simulink model "dynamics_kinematics"  (Simulink 7.9)
settings: Solver=ode15s  StartTime=0.0  StopTime=10.0  RelTol=1e-3
values from neighbouring files (symbols this model uses):
  current_s = [0,1,0,0,0,0, 0,0,0,0,0,0] * 0    [kinematic_parameters.m]
  initial_ee_eta = zeros(1,6)    [kinematic_parameters.m]
  initial_eta = [0,0,0,0,0,0]    [kinematic_parameters.m]
  initial_q = [0,65*d2r,-(65+90)*d2r,90*d2r,-90*d2r,0]    [kinematic_parameters.m]
  inner_motion_vec = [0,0,0,0,0,1,0,0,0,0,0,0]    [kinematic_parameters.m]
  K_i = diag([1,1,1,1,1,1,   1,1,1,1,1,1])*0.5 * 0    [kinematic_parameters.m]
  K_p = diag([1,1,1,1,1,1,   1,1,1,1,1,1])    [kinematic_parameters.m]
  v_ee_c = [0.1,0,0,0,0,0]    [kinematic_parameters.m]
libraries: simulink x1
settings Model: Creator=simena  LastModifiedBy=simena  SimulationMode=accelerator
settings OptimizationCC: EfficientMapNaN2IntZero=off
settings HardwareCC: TargetIntDivRoundTo=Zero  TargetEndianess=LittleEndian  TargetHWDeviceType=MATLAB Host  ProdEqTarget=off
settings CodeAppCC: MaxIdLength=128
settings GRTTargetCC: CombineOutputUpdateFcns=off  GRTInterface=on

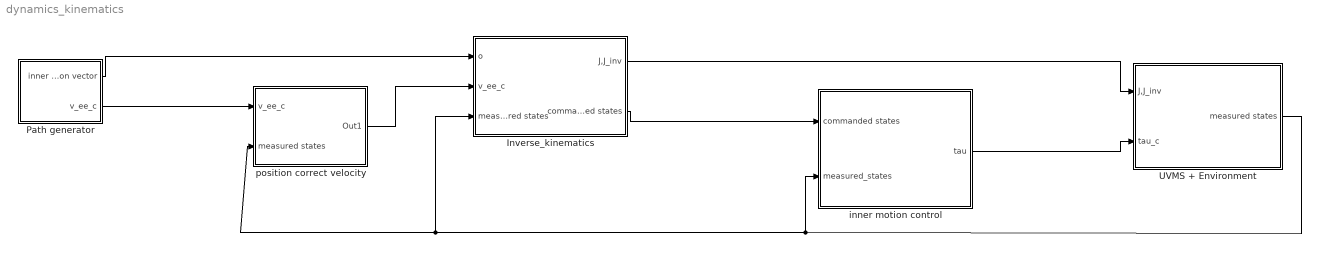
== system dynamics_kinematics ==
  "Inverse_kinematics " : Subsystem
  Path generator : Subsystem
  UVMS + Environment : Subsystem
  inner motion control : Subsystem
  position correct velocity : Subsystem
  wires:
  inner motion control/1(tau) -> UVMS + Environment/2(tau_c)
  UVMS + Environment/1(measured states) -> inner motion control/2(measured_states), "Inverse_kinematics "/3(measured states), position correct velocity/2(measured states)
  "Inverse_kinematics "/2(commanded states) -> inner motion control/1(commanded states)
  Path generator/1(inner motion vector) -> "Inverse_kinematics "/1(o)
  Path generator/2(v_ee_c) -> position correct velocity/1(v_ee_c)
  position correct velocity/1(Out1) -> "Inverse_kinematics "/2(v_ee_c)
  "Inverse_kinematics "/1(J,J_inv) -> UVMS + Environment/1(J,J_inv)

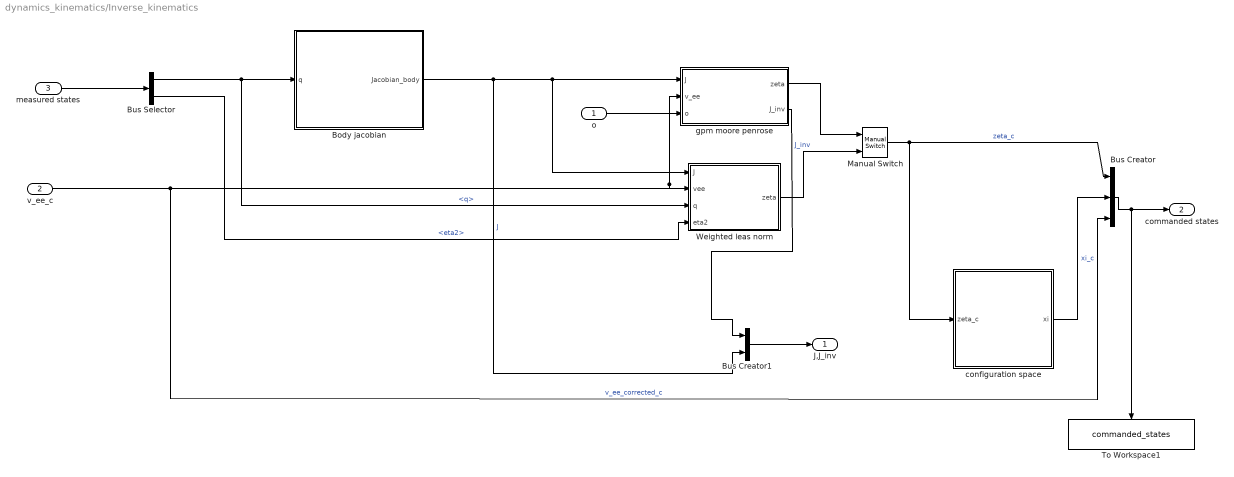
== system dynamics_kinematics/Inverse_kinematics  ==
  o : Inport
  v_ee_c : Inport  Port=2
  measured states : Inport  Port=3
  Body jacobian : MATLAB Function  TreatAsAtomicUnit=on
  Bus Creator : BusCreator  Inputs=3
  Bus Creator1 : BusCreator  Inputs=2
  Bus Selector : BusSelector  OutputSignals=xi.q,xi.eta2
  Manual Switch : simulink/Signal Routing/Manual Switch  sw=0  action=0  varsize=off
  To Workspace1 : ToWorkspace  VariableName=commanded_states  SampleTime=-1  SaveFormat=Timeseries
  Weighted leas norm : MATLAB Function  TreatAsAtomicUnit=on
  configuration space : Subsystem
  gpm moore penrose : Subsystem
  J,J_inv : Outport
  commanded states : Outport  Port=2
  wires:
  gpm moore penrose/1(zeta) -> Manual Switch/1
  Weighted leas norm/1(zeta) -> Manual Switch/2
  Manual Switch/1 -> configuration space/1(zeta_c), Bus Creator/1  "zeta_c"
  measured states/1 -> Bus Selector/1
  Bus Selector/1 -> Body jacobian/1(q), Weighted leas norm/3(q)  "<q>"
  Body jacobian/1(Jacobian_body) -> gpm moore penrose/1(J), Weighted leas norm/1(J), Bus Creator1/2  "J"
  Bus Selector/2 -> Weighted leas norm/4(eta2)  "<eta2>"
  v_ee_c/1 -> gpm moore penrose/2(v_ee), Weighted leas norm/2(vee), Bus Creator/3  "v_ee_corrected_c"
  o/1 -> gpm moore penrose/3(o)
  configuration space/1(xi) -> Bus Creator/2  "xi_c"
  Bus Creator/1 -> commanded states/1, To Workspace1/1
  Bus Creator1/1 -> J,J_inv/1
  gpm moore penrose/2(J_inv) -> Bus Creator1/1  "J_inv"

== system dynamics_kinematics/Path generator ==
  Bus Creator : BusCreator  Inputs=2
  Inner motion vector : Constant  Value=inner_motion_vec
  To Workspace : ToWorkspace  VariableName=path_c  SampleTime=-1  SaveFormat=Timeseries
  commanded trajectory : Subsystem
  v_ee_command : Constant  Value=v_ee_c
  inner motion vector : Outport
  v_ee_c : Outport  Port=2
  wires:
  Inner motion vector/1 -> inner motion vector/1
  v_ee_command/1 -> commanded trajectory/1(v_ee), Bus Creator/1  "v_ee_c"
  commanded trajectory/1(ee_pose) -> Bus Creator/2
  Bus Creator/1 -> v_ee_c/1, To Workspace/1

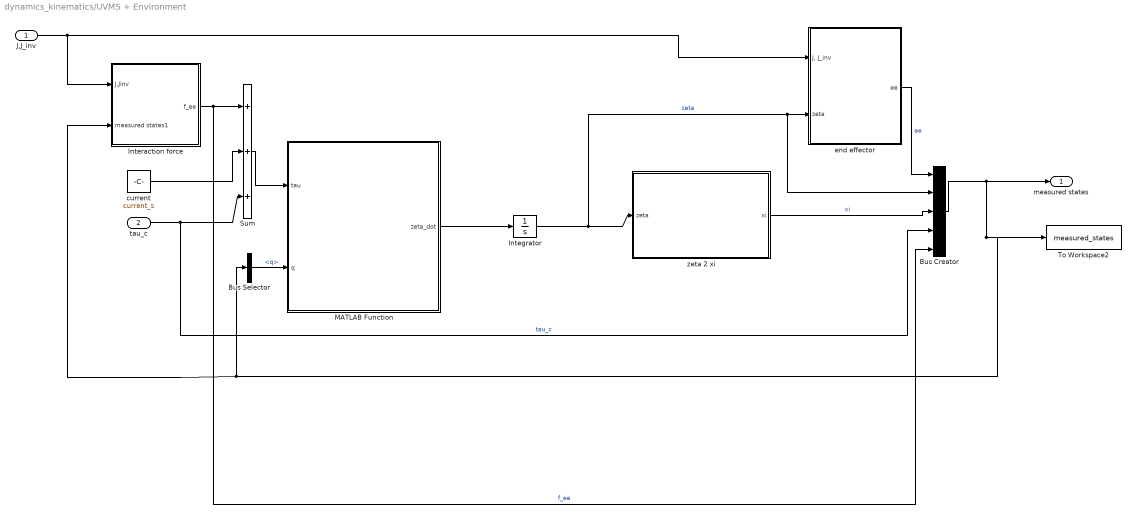
== system dynamics_kinematics/UVMS + Environment ==
  J,J_inv : Inport
  tau_c : Inport  Port=2
  Bus Creator : BusCreator  Inputs=5
  Bus Selector : BusSelector  OutputSignals=xi.q
  Integrator : Integrator
  Interaction force : Subsystem
  MATLAB Function : MATLAB Function  TreatAsAtomicUnit=on
  Sum : Sum  Inputs=+++
  To Workspace2 : ToWorkspace  VariableName=measured_states  SampleTime=-1  SaveFormat=Timeseries
  current : Constant  Value=current_s
  end effector : Subsystem
  zeta 2 xi : Subsystem
  measured states : Outport
  wires:
  MATLAB Function/1(zeta_dot) -> Integrator/1
  Integrator/1 -> zeta 2 xi/1(zeta), end effector/2(zeta), Bus Creator/2  "zeta"
  zeta 2 xi/1(xi) -> Bus Creator/3  "xi"
  Bus Selector/1 -> MATLAB Function/2(q)  "<q>"
  J,J_inv/1 -> end effector/1("J, J_inv"), Interaction force/1(J,Jinv)
  Bus Creator/1 -> measured states/1, To Workspace2/1, Bus Selector/1, Interaction force/2(measured states1)
  end effector/1(ee) -> Bus Creator/1  "ee"
  Sum/1 -> MATLAB Function/1(tau)
  current/1 -> Sum/2
  tau_c/1 -> Sum/3, Bus Creator/4  "tau_c"
  Interaction force/1(f_ee) -> Sum/1, Bus Creator/5  "f_ee"

== system dynamics_kinematics/inner motion control ==
  commanded states : Inport
  measured_states : Inport  Port=2
  Inertia M : MATLAB Function  TreatAsAtomicUnit=on
  Product : Product  Multiplication=Matrix(*)  RndMeth=Zero
  Subsystem : Subsystem
  tau : Outport
  wires:
  Inertia M/1(M) -> Product/1
  Product/1 -> tau/1
  commanded states/1 -> Subsystem/1(commanded states)
  measured_states/1 -> Subsystem/2(measured_states)
  Subsystem/1(q) -> Inertia M/1(q)
  Subsystem/2(a) -> Product/2

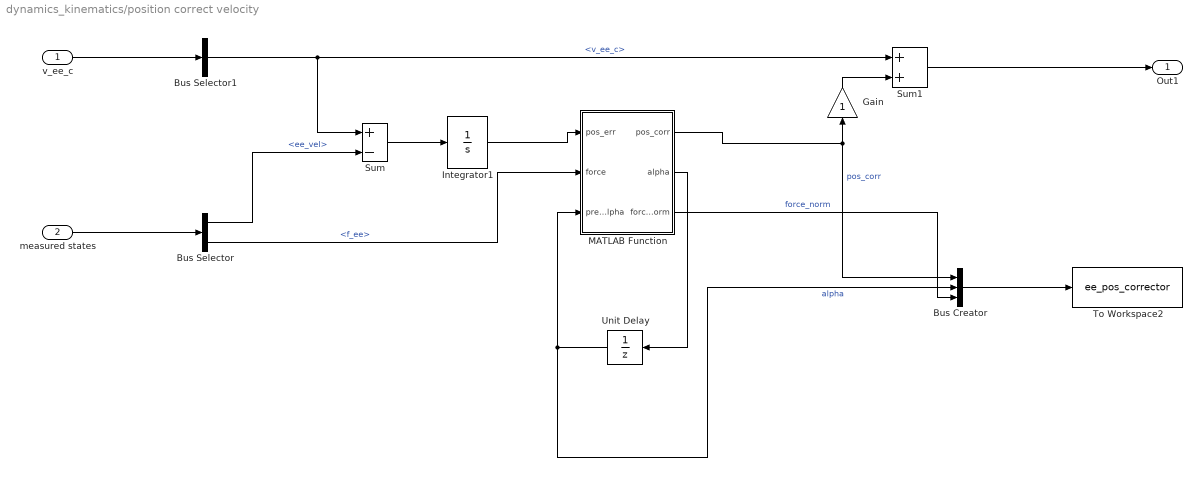
== system dynamics_kinematics/position correct velocity ==
  v_ee_c : Inport
  measured states : Inport  Port=2
  Bus Creator : BusCreator  Inputs=3
  Bus Selector : BusSelector  OutputSignals=ee.ee_vel,f_ee
  Bus Selector1 : BusSelector  OutputSignals=v_ee_c
  Gain : Gain
  Integrator1 : Integrator
  MATLAB Function : MATLAB Function  TreatAsAtomicUnit=on
  Sum : Sum  Inputs=+-
  Sum1 : Sum
  To Workspace2 : ToWorkspace  VariableName=ee_pos_corrector  SampleTime=-1  SaveFormat=Timeseries
  Unit Delay : UnitDelay  X0=1  SampleTime=-1
  Out1 : Outport
  wires:
  Sum1/1 -> Out1/1
  MATLAB Function/1(pos_corr) -> Bus Creator/1, Gain/1  "pos_corr"
  measured states/1 -> Bus Selector/1
  v_ee_c/1 -> Bus Selector1/1
  Bus Selector1/1 -> Sum1/1, Sum/1  "<v_ee_c>"
  Sum/1 -> Integrator1/1
  Bus Selector/2 -> MATLAB Function/2(force)  "<f_ee>"
  Bus Selector/1 -> Sum/2  "<ee_vel>"
  Integrator1/1 -> MATLAB Function/1(pos_err)
  MATLAB Function/2(alpha) -> Unit Delay/1
  Unit Delay/1 -> MATLAB Function/3(prev_alpha), Bus Creator/2  "alpha"
  Bus Creator/1 -> To Workspace2/1
  MATLAB Function/3(force_norm) -> Bus Creator/3  "force_norm"
  Gain/1 -> Sum1/2

== system dynamics_kinematics/Inverse_kinematics /configuration space ==
  zeta_c : Inport
  Bus Creator : BusCreator  Inputs=3
  quasi velocity 2 generalized rates : Subsystem
  xi : Outport
  wires:
  quasi velocity 2 generalized rates/1(position vehicle) -> Bus Creator/1  "eta1"
  quasi velocity 2 generalized rates/2(attitude vehicle) -> Bus Creator/2  "eta2"
  quasi velocity 2 generalized rates/3(q) -> Bus Creator/3  "q"
  Bus Creator/1 -> xi/1
  zeta_c/1 -> quasi velocity 2 generalized rates/1(zeta)

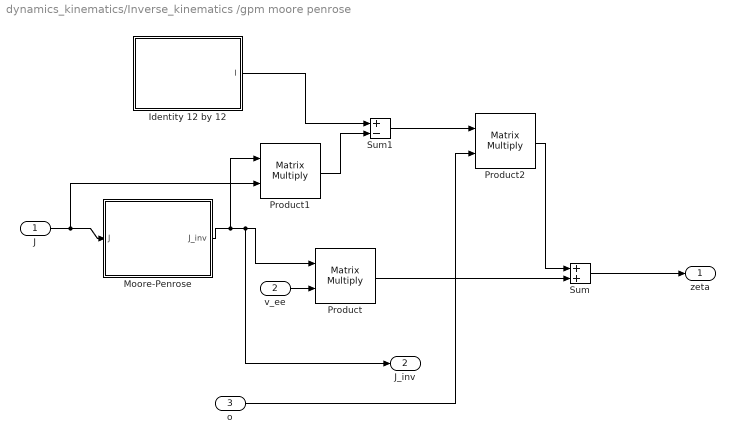
== system dynamics_kinematics/Inverse_kinematics /gpm moore penrose ==
  J : Inport
  v_ee : Inport  Port=2
  o : Inport  Port=3
  Identity 12 by 12 : MATLAB Function  TreatAsAtomicUnit=on
  Moore-Penrose : MATLAB Function  TreatAsAtomicUnit=on
  Product : Product  Multiplication=Matrix(*)  RndMeth=Zero
  Product1 : Product  Multiplication=Matrix(*)  RndMeth=Zero
  Product2 : Product  Multiplication=Matrix(*)  RndMeth=Zero
  Sum : Sum
  Sum1 : Sum  Inputs=+-
  zeta : Outport
  J_inv : Outport  Port=2
  wires:
  J/1 -> Product1/2, Moore-Penrose/1(J)
  Moore-Penrose/1(J_inv) -> Product1/1, Product/1, J_inv/1
  Product/1 -> Sum/2
  Identity 12 by 12/1(I) -> Sum1/1
  Product1/1 -> Sum1/2
  Sum1/1 -> Product2/1
  Product2/1 -> Sum/1
  v_ee/1 -> Product/2
  Sum/1 -> zeta/1
  o/1 -> Product2/2

== system dynamics_kinematics/Path generator/commanded trajectory ==
  v_ee : Inport
  Bus Creator : BusCreator  Inputs=2
  Demux : Demux  Outputs=2
  Integrator : Integrator  InitialCondition=initial_ee_eta
  body2eulervel : MATLAB Function  TreatAsAtomicUnit=on
  ee_pose : Outport
  wires:
  v_ee/1 -> body2eulervel/1(ee_velocity)
  body2eulervel/1(ee_rates) -> Integrator/1
  Integrator/1 -> Demux/1
  Demux/1 -> Bus Creator/1  "ee_pos"
  Demux/2 -> body2eulervel/2(euler_angles_ee), Bus Creator/2  "ee_angle"
  Bus Creator/1 -> ee_pose/1  "ee_pose"

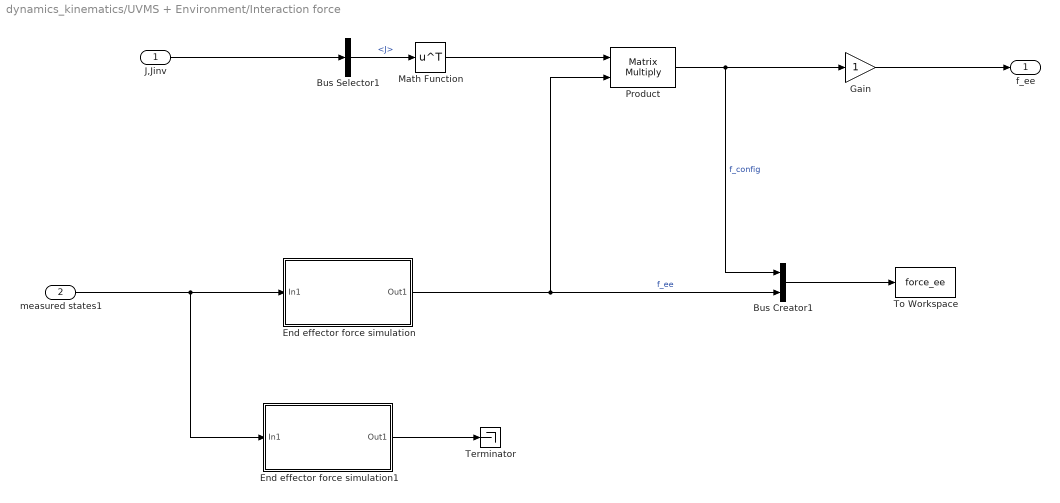
== system dynamics_kinematics/UVMS + Environment/Interaction force ==
  J,Jinv : Inport
  measured states1 : Inport  Port=2
  Bus Creator1 : BusCreator  Inputs=2
  Bus Selector1 : BusSelector  OutputSignals=J
  End effector force simulation : Subsystem
  End effector force simulation1 : Subsystem
  Gain : Gain
  Math Function : Math  Operator=transpose  SaturateOnIntegerOverflow=on
  Product : Product  Multiplication=Matrix(*)  RndMeth=Zero
  Terminator : Terminator
  To Workspace : ToWorkspace  VariableName=force_ee  SampleTime=-1  SaveFormat=Timeseries
  f_ee : Outport
  wires:
  measured states1/1 -> End effector force simulation/1(In1), End effector force simulation1/1(In1)
  J,Jinv/1 -> Bus Selector1/1
  Bus Selector1/1 -> Math Function/1  "<J>"
  Math Function/1 -> Product/1
  End effector force simulation/1(Out1) -> Product/2, Bus Creator1/2  "f_ee"
  Product/1 -> Bus Creator1/1, Gain/1  "f_config"
  Bus Creator1/1 -> To Workspace/1
  Gain/1 -> f_ee/1
  End effector force simulation1/1(Out1) -> Terminator/1

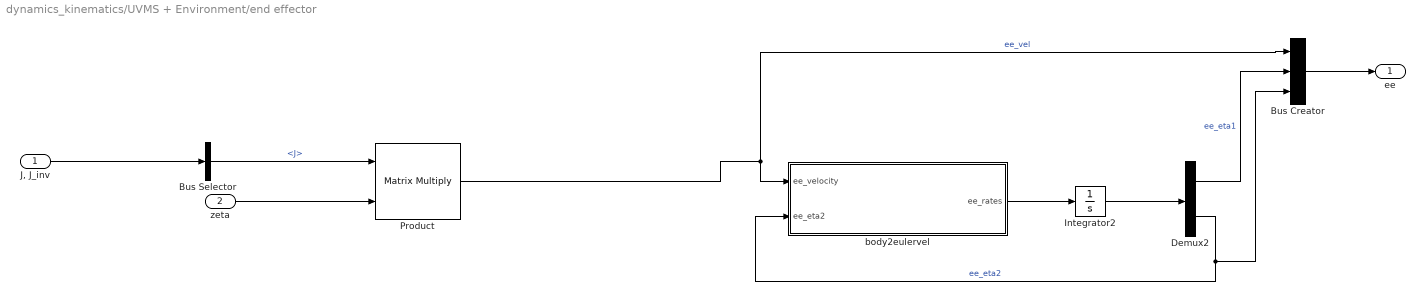
== system dynamics_kinematics/UVMS + Environment/end effector ==
  "J, J_inv" : Inport
  zeta : Inport  Port=2
  Bus Creator : BusCreator  Inputs=3
  Bus Selector : BusSelector  OutputSignals=J
  Demux2 : Demux  Outputs=2
  Integrator2 : Integrator  InitialCondition=initial_ee_eta
  Product : Product  Multiplication=Matrix(*)  RndMeth=Zero
  body2eulervel : MATLAB Function  TreatAsAtomicUnit=on
  ee : Outport
  wires:
  zeta/1 -> Product/2
  Demux2/2 -> body2eulervel/2(ee_eta2), Bus Creator/3  "ee_eta2"
  Integrator2/1 -> Demux2/1
  body2eulervel/1(ee_rates) -> Integrator2/1
  Product/1 -> body2eulervel/1(ee_velocity), Bus Creator/1  "ee_vel"
  Demux2/1 -> Bus Creator/2  "ee_eta1"
  Bus Creator/1 -> ee/1
  "J, J_inv"/1 -> Bus Selector/1
  Bus Selector/1 -> Product/1  "<J>"

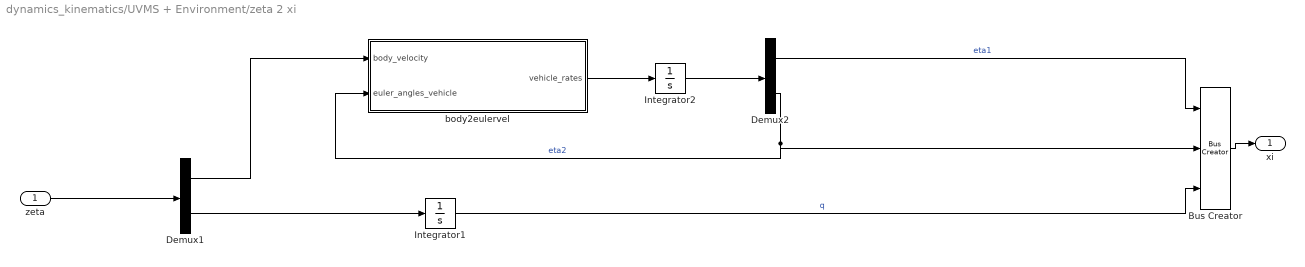
== system dynamics_kinematics/UVMS + Environment/zeta 2 xi ==
  zeta : Inport
  Bus Creator : BusCreator  Inputs=3
  Demux1 : Demux  Outputs=2
  Demux2 : Demux  Outputs=2
  Integrator1 : Integrator  InitialCondition=initial_q
  Integrator2 : Integrator  InitialCondition=initial_eta
  body2eulervel : MATLAB Function  TreatAsAtomicUnit=on
  xi : Outport
  wires:
  Demux2/1 -> Bus Creator/1  "eta1"
  Demux2/2 -> body2eulervel/2(euler_angles_vehicle), Bus Creator/2  "eta2"
  Integrator2/1 -> Demux2/1
  body2eulervel/1(vehicle_rates) -> Integrator2/1
  Integrator1/1 -> Bus Creator/3  "q"
  Demux1/1 -> body2eulervel/1(body_velocity)
  Demux1/2 -> Integrator1/1
  zeta/1 -> Demux1/1
  Bus Creator/1 -> xi/1

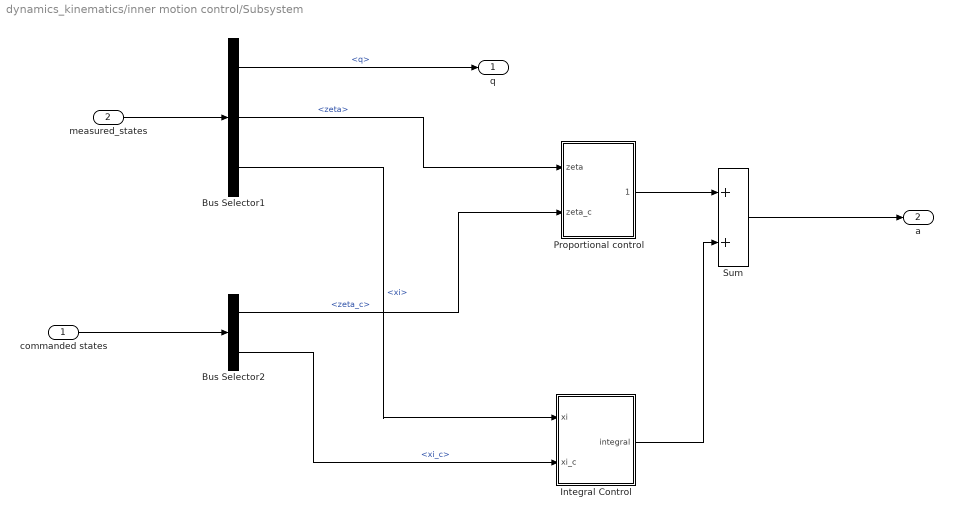
== system dynamics_kinematics/inner motion control/Subsystem ==
  commanded states : Inport
  measured_states : Inport  Port=2
  Bus Selector1 : BusSelector  OutputSignals=xi.q,zeta,xi
  Bus Selector2 : BusSelector  OutputSignals=zeta_c,xi_c
  Integral Control : Subsystem
  Proportional control : Subsystem
  Sum : Sum
  q : Outport
  a : Outport  Port=2
  wires:
  measured_states/1 -> Bus Selector1/1
  commanded states/1 -> Bus Selector2/1
  Bus Selector1/2 -> Proportional control/1(zeta)  "<zeta>"
  Bus Selector2/1 -> Proportional control/2(zeta_c)  "<zeta_c>"
  Bus Selector1/1 -> q/1  "<q>"
  Proportional control/1(proportional) -> Sum/1
  Bus Selector1/3 -> Integral Control/1(xi)  "<xi>"
  Bus Selector2/2 -> Integral Control/2(xi_c)  "<xi_c>"
  Integral Control/1(integral) -> Sum/2
  Sum/1 -> a/1

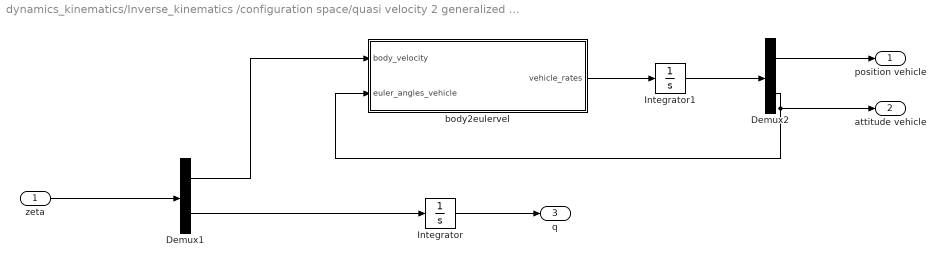
== system dynamics_kinematics/Inverse_kinematics /configuration space/quasi velocity 2 generalized rates ==
  zeta : Inport
  Demux1 : Demux  Outputs=2
  Demux2 : Demux  Outputs=2
  Integrator : Integrator  InitialCondition=initial_q
  Integrator1 : Integrator  InitialCondition=initial_eta
  body2eulervel : MATLAB Function  TreatAsAtomicUnit=on
  position vehicle : Outport
  attitude vehicle : Outport  Port=2
  q : Outport  Port=3
  wires:
  zeta/1 -> Demux1/1
  Demux1/2 -> Integrator/1
  Demux1/1 -> body2eulervel/1(body_velocity)
  Integrator/1 -> q/1
  body2eulervel/1(vehicle_rates) -> Integrator1/1
  Integrator1/1 -> Demux2/1
  Demux2/2 -> body2eulervel/2(euler_angles_vehicle), attitude vehicle/1
  Demux2/1 -> position vehicle/1

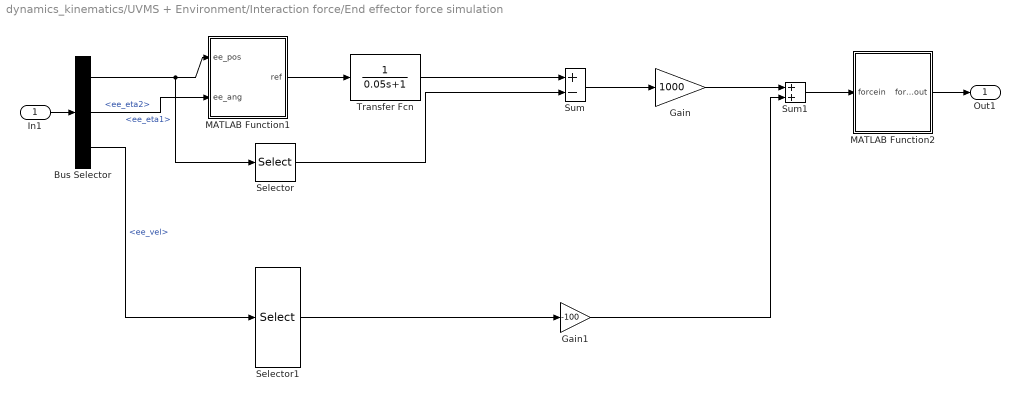
== system dynamics_kinematics/UVMS + Environment/Interaction force/End effector force simulation ==
  In1 : Inport
  Bus Selector : BusSelector  OutputSignals=ee.ee_eta1,ee.ee_eta2,ee.ee_vel
  Gain : Gain  Gain=1000
  Gain1 : Gain  Gain=-100
  MATLAB Function1 : MATLAB Function  TreatAsAtomicUnit=on
  MATLAB Function2 : MATLAB Function  TreatAsAtomicUnit=on
  Selector : Selector  InputPortWidth=3  IndexOptions=Index vector (dialog)  Indices=[2]  OutputSizes=1
  Selector1 : Selector  InputPortWidth=6  IndexOptions=Index vector (dialog)  Indices=2  OutputSizes=1
  Sum : Sum  Inputs=+-
  Sum1 : Sum
  Transfer Fcn : TransferFcn  Denominator=[0.05 1]
  Out1 : Outport
  wires:
  In1/1 -> Bus Selector/1
  Bus Selector/1 -> MATLAB Function1/1(ee_pos), Selector/1  "<ee_eta1>"
  MATLAB Function1/1(ref) -> Transfer Fcn/1
  Transfer Fcn/1 -> Sum/1
  Sum/1 -> Gain/1
  Gain/1 -> Sum1/1
  Sum1/1 -> MATLAB Function2/1(forcein)
  Bus Selector/3 -> Selector1/1  "<ee_vel>"
  Bus Selector/2 -> MATLAB Function1/2(ee_ang)  "<ee_eta2>"
  Selector/1 -> Sum/2
  Selector1/1 -> Gain1/1
  Gain1/1 -> Sum1/2
  MATLAB Function2/1(forceout) -> Out1/1

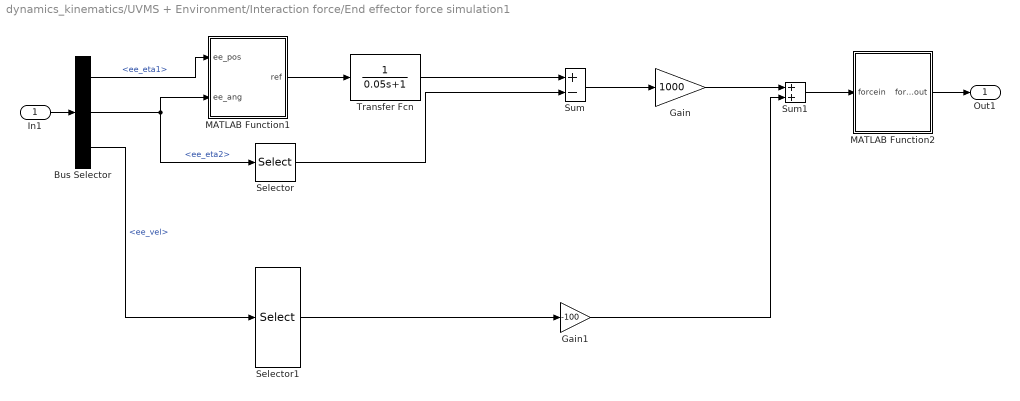
== system dynamics_kinematics/UVMS + Environment/Interaction force/End effector force simulation1 ==
  In1 : Inport
  Bus Selector : BusSelector  OutputSignals=ee.ee_eta1,ee.ee_eta2,ee.ee_vel
  Gain : Gain  Gain=1000
  Gain1 : Gain  Gain=-100
  MATLAB Function1 : MATLAB Function  TreatAsAtomicUnit=on
  MATLAB Function2 : MATLAB Function  TreatAsAtomicUnit=on
  Selector : Selector  InputPortWidth=3  IndexOptions=Index vector (dialog)  Indices=[3]  OutputSizes=1
  Selector1 : Selector  InputPortWidth=6  IndexOptions=Index vector (dialog)  Indices=6  OutputSizes=1
  Sum : Sum  Inputs=+-
  Sum1 : Sum
  Transfer Fcn : TransferFcn  Denominator=[0.05 1]
  Out1 : Outport
  wires:
  In1/1 -> Bus Selector/1
  Bus Selector/1 -> MATLAB Function1/1(ee_pos)  "<ee_eta1>"
  MATLAB Function1/1(ref) -> Transfer Fcn/1
  Transfer Fcn/1 -> Sum/1
  Sum/1 -> Gain/1
  Gain/1 -> Sum1/1
  Sum1/1 -> MATLAB Function2/1(forcein)
  Bus Selector/3 -> Selector1/1  "<ee_vel>"
  Bus Selector/2 -> Selector/1, MATLAB Function1/2(ee_ang)  "<ee_eta2>"
  Selector/1 -> Sum/2
  Selector1/1 -> Gain1/1
  Gain1/1 -> Sum1/2
  MATLAB Function2/1(forceout) -> Out1/1

== system dynamics_kinematics/inner motion control/Subsystem/Integral Control ==
  xi : Inport
  xi_c : Inport  Port=2
  Bus to Vector : BusToVector
  Bus to Vector1 : BusToVector
  Gain : Gain  Gain=K_i  Multiplication=Matrix(K*u)
  Sum1 : Sum  Inputs=+-
  integral : Outport
  wires:
  Sum1/1 -> Gain/1
  xi_c/1 -> Bus to Vector/1
  Bus to Vector/1 -> Sum1/1
  xi/1 -> Bus to Vector1/1
  Bus to Vector1/1 -> Sum1/2
  Gain/1 -> integral/1

== system dynamics_kinematics/inner motion control/Subsystem/Proportional control ==
  zeta : Inport
  zeta_c : Inport  Port=2
  Gain : Gain  Gain=K_p  Multiplication=Matrix(K*u)
  Sum : Sum  Inputs=-+
  proportional : Outport
  wires:
  Sum/1 -> Gain/1
  Gain/1 -> proportional/1
  zeta/1 -> Sum/1
  zeta_c/1 -> Sum/2

== matlab function Inverse_kinematics /gpm moore penrose/Identity 12 by 12 ==
  data: I output double
function I = Identity_mat()
    %#codegen
    I=eye(12);
end

== matlab function Inverse_kinematics /Body jacobian ==
  data: q input double; Jacobian_body output double
function Jacobian_body = fcn(q)
    %#codegen
    Jacobian_body=zeros(6,12);
    coder.extrinsic('body_jacobian');
    newq=zeros(1,6);
    newq=q;
    Jacobian_body=body_jacobian(newq);
end

== matlab function Inverse_kinematics /configuration space/quasi velocity 2 generalized rates/body2eulervel ==
  data: body_velocity input double; vehicle_rates output double; euler_angles_vehicle input double
function vehicle_rates = fcn(body_velocity, euler_angles_vehicle)                       
    %#codegen
    coder.extrinsic('analytical_jacobian');
    J=analytical_jacobian(euler_angles_vehicle);

    vehicle_rates = zeros(6,1);
    vehicle_rates=J*body_velocity;
end

== matlab function Inverse_kinematics /gpm moore penrose/Moore-Penrose ==
  data: J input double; J_inv output double
function J_inv = moore_penrose(J)
    %#codegen
    coder.extrinsic('mp_inv');
    
    J_inv=zeros(12,6);
    J_inv = mp_inv(J);
        
end

== matlab function UVMS + Environment/end effector/body2eulervel ==
  data: ee_velocity input double; ee_rates output double; ee_eta2 input double
function ee_rates = fcn(ee_velocity, ee_eta2)                       
    %#codegen
    coder.extrinsic('analytical_jacobian');
    J=analytical_jacobian(ee_eta2);

    ee_rates = zeros(6,1);
    ee_rates=J*ee_velocity;
end

== matlab function Inverse_kinematics /Weighted leas norm ==
  data: J input double; zeta output double; vee input double; q input double; eta2 input double
function zeta = wln(J,vee,q, eta2)
%#codegen
    coder.extrinsic('wln_m');
    J_inv=zeros(12,6);
    J_inv=wln_m(J,q,eta2);    
    
    zeta = J_inv(1:12,1:6)*vee;
end

== matlab function Path generator/commanded trajectory/body2eulervel ==
  data: ee_velocity input double; ee_rates output double; euler_angles_ee input double
function ee_rates = fcn(ee_velocity, euler_angles_ee)                       
    %#codegen
    coder.extrinsic('analytical_jacobian');
    J=analytical_jacobian(euler_angles_ee);

    ee_rates = zeros(6,1);
    ee_rates=J*ee_velocity;
end

== matlab function UVMS + Environment/Interaction force/End effector force simulation/MATLAB Function2 ==
  data: forceout output double; forcein input double
function forceout = fcn(forcein)
    %#codegen
    forceout= zeros(6,1);
    forceout(2) = forcein;
    
    
end

== matlab function UVMS + Environment/MATLAB Function ==
  data: tau input double; zeta_dot output double; q input double
function zeta_dot  = tau2acceleration(tau,q)
    %#codegen
    coder.extrinsic('getInertia')
    M=zeros(12,12);
    M=getInertia(q);
    m_inv=zeros(12,12);
    m_inv=inv(M);
    zeta_dot = m_inv*tau ;
end

== matlab function inner motion control/Inertia M ==
  data: M output double; q input double
function M = tau2acceleration(q)
    %#codegen
    coder.extrinsic('getInertia')
    M=zeros(12,12);
    M=getInertia(q);
end

== matlab function UVMS + Environment/zeta 2 xi/body2eulervel ==
  data: body_velocity input double; vehicle_rates output double; euler_angles_vehicle input double
function vehicle_rates = fcn(body_velocity, euler_angles_vehicle)                       
    %#codegen
    coder.extrinsic('analytical_jacobian');
    J=analytical_jacobian(euler_angles_vehicle);

    vehicle_rates = zeros(6,1);
    vehicle_rates=J*body_velocity;
end

== matlab function UVMS + Environment/Interaction force/End effector force simulation1/MATLAB Function1 ==
  data: ref output double; ee_pos input double; ee_ang input double
function ref = fcn(ee_pos,ee_ang)
    %#codegen
    ref = ee_ang(3);
    if ee_pos(1)>1.5 & ee_pos(1)<1.52
       ref=(pi/180)*10*abs(ee_pos(1) - 1.5)*50; 
    elseif ee_pos(1)>1.52
        ref=(pi/180)*10;
    end
  
    
end

== matlab function UVMS + Environment/Interaction force/End effector force simulation/MATLAB Function1 ==
  data: ref output double; ee_pos input double; ee_ang input double
function ref = fcn(ee_pos,ee_ang)
    %#codegen
    ref = ee_pos(2);
    if ee_pos(1)>=1.5 
        ref=0.4*(ee_pos(1)-1.5);
    end
      
end

== matlab function position correct velocity/MATLAB Function ==
  data: pos_err input double; pos_corr output double; force input double; prev_alpha input double; alpha output double; force_norm output double
function [pos_corr, alpha,force_norm]  = fcn(pos_err,force,prev_alpha)
%#codegen
    %global alpha;
    alpha=ones(1,1);
    
    force_n = norm(force);
    reset=0;
    
    if prev_alpha == 0
        alpha =0;
    elseif force_n < 0.1
        alpha = 1;
    elseif force_n < 0.3
        alpha = 1-(force_n-0.1)*3;
    else
        reset=1;
        alpha = 0;
    end
    alpha=1;
    K_pos_correction = zeros(6,6);
    K_pos_correction = diag([0,alpha*0.5,alpha*0.5 ,0,alpha*0.4,alpha*0.4])*10;
    pos_corr=zeros(6,1);
    pos_corr = K_pos_correction * pos_err;
    force_norm=1;
    force_norm=force_n;
end

== matlab function UVMS + Environment/Interaction force/End effector force simulation1/MATLAB Function2 ==
  data: forceout output double; forcein input double
function forceout = fcn(forcein)
    %#codegen
    forceout= zeros(6,1);
    forceout(6) = forcein;
    
    
end
